simulink model "FSModem_FPGA"  (R2017b)
settings: Solver=FixedStepDiscrete  StartTime=0.0  StopTime=10.0  RelTol=1e-3
InitFcn:
  | theta = 0:pi/4:(2*pi)-(pi/4);
  | Fs_8 = cos(theta) +i*sin(theta);
  | sample_time = 1/1e6;
undefined symbols (not defined in the file): i
libraries: hdlsllib x2
settings Model: DataTypeOverride=Off  Creator=ppradhan  LastModifiedBy=ppradhan
settings DataIOCC: SaveOutput=off  SaveTime=off
settings OptimizationCC: BlockReduction=off  ConditionallyExecuteInputs=off  DefaultParameterBehavior=Inlined
settings DebuggingCC: AlgebraicLoopMsg=error  SingleTaskRateTransMsg=error  StrictBusMsg=ErrorOnBusTreatedAsVector
settings HardwareCC: ProdBitPerPointer=32  ProdBitPerSizeT=32  ProdBitPerPtrDiffT=32  ProdLargestAtomicFloat=None  ProdIntDivRoundTo=Undefined  ProdEndianess=Unspecified  ProdWordSize=32  ProdHWDeviceType=ASIC/FPGA->ASIC/FPGA  ProdEqTarget=off
settings CodeAppCC: StateflowObjectComments=on

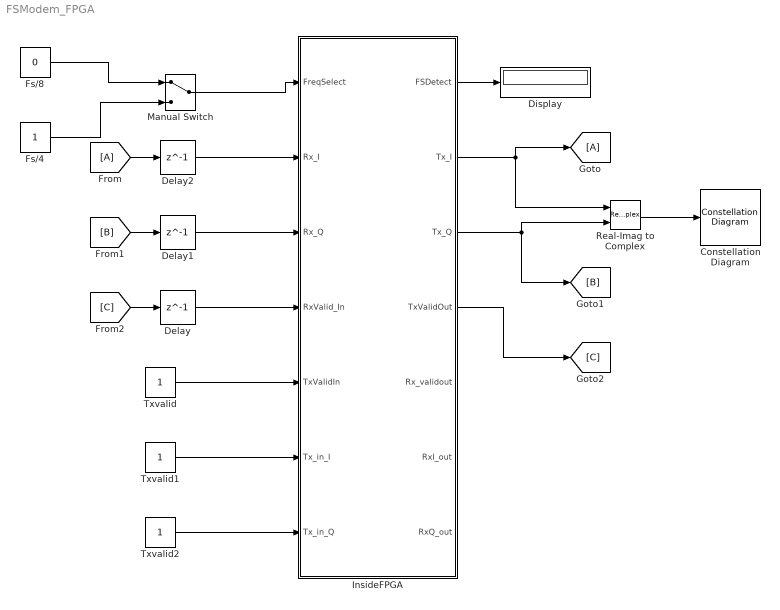
== system FSModem_FPGA ==
  Constellation Diagram : ConstellationDiagram
  Delay : Delay  DelayLength=1
  Delay1 : Delay  DelayLength=1
  Delay2 : Delay  DelayLength=1
  Display : Display
  Fs/4 : Constant  OutDataTypeStr=boolean  SampleTime=sample_time
  Fs/8 : Constant  Value=0  OutDataTypeStr=boolean  SampleTime=sample_time
  InsideFPGA : Subsystem  TreatAsAtomicUnit=on
  Manual Switch : ManualSwitch
  Real-Imag to Complex : RealImagToComplex
  Txvalid : Constant  OutDataTypeStr=boolean  SampleTime=sample_time
  Txvalid1 : Constant  OutDataTypeStr=int16  SampleTime=sample_time
  Txvalid2 : Constant  OutDataTypeStr=int16  SampleTime=sample_time
  wires:
  InsideFPGA/1(FSDetect) -> Display/1
  InsideFPGA/2(Tx_I) -> Real-Imag to Complex/1, [A]
  [A] -> Delay2/1
  InsideFPGA/3(Tx_Q) -> [B], Real-Imag to Complex/2
  [B] -> Delay1/1
  InsideFPGA/4(TxValidOut) -> [C]
  [C] -> Delay/1
  Delay/1 -> InsideFPGA/4(RxValid_In)
  Delay1/1 -> InsideFPGA/3(Rx_Q)
  Delay2/1 -> InsideFPGA/2(Rx_I)
  Real-Imag to Complex/1 -> Constellation Diagram/1
  Fs/8/1 -> Manual Switch/1
  Fs/4/1 -> Manual Switch/2
  Manual Switch/1 -> InsideFPGA/1(FreqSelect)
  Txvalid/1 -> InsideFPGA/5(TxValidIn)
  Txvalid1/1 -> InsideFPGA/6(Tx_in_I)
  Txvalid2/1 -> InsideFPGA/7(Tx_in_Q)

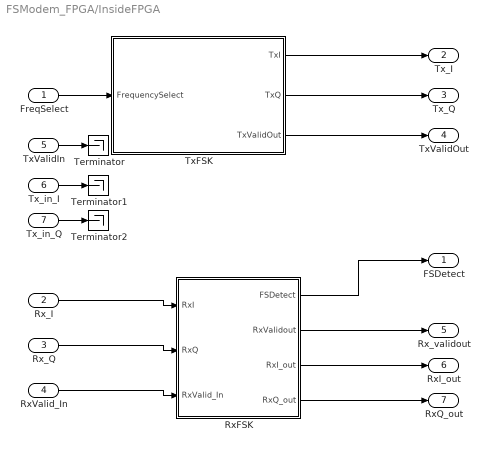
== system FSModem_FPGA/InsideFPGA ==
  FreqSelect : Inport
  Rx_I : Inport  Port=2
  Rx_Q : Inport  Port=3
  RxValid_In : Inport  Port=4
  TxValidIn : Inport  Port=5
  Tx_in_I : Inport  Port=6
  Tx_in_Q : Inport  Port=7
  RxFSK : Subsystem
  Terminator : Terminator
  Terminator1 : Terminator
  Terminator2 : Terminator
  TxFSK : Subsystem
  FSDetect : Outport
  Tx_I : Outport  Port=2
  Tx_Q : Outport  Port=3
  TxValidOut : Outport  Port=4
  Rx_validout : Outport  Port=5
  RxI_out : Outport  Port=6
  RxQ_out : Outport  Port=7
  wires:
  FreqSelect/1 -> TxFSK/1(FrequencySelect)
  RxFSK/1(FSDetect) -> FSDetect/1
  Rx_I/1 -> RxFSK/1(RxI)
  Rx_Q/1 -> RxFSK/2(RxQ)
  RxValid_In/1 -> RxFSK/3(RxValid_In)
  TxFSK/3(TxValidOut) -> TxValidOut/1
  TxFSK/1(TxI) -> Tx_I/1
  TxFSK/2(TxQ) -> Tx_Q/1
  RxFSK/2(RxValidout) -> Rx_validout/1
  TxValidIn/1 -> Terminator/1
  Tx_in_I/1 -> Terminator1/1
  Tx_in_Q/1 -> Terminator2/1
  RxFSK/3(RxI_out) -> RxI_out/1
  RxFSK/4(RxQ_out) -> RxQ_out/1

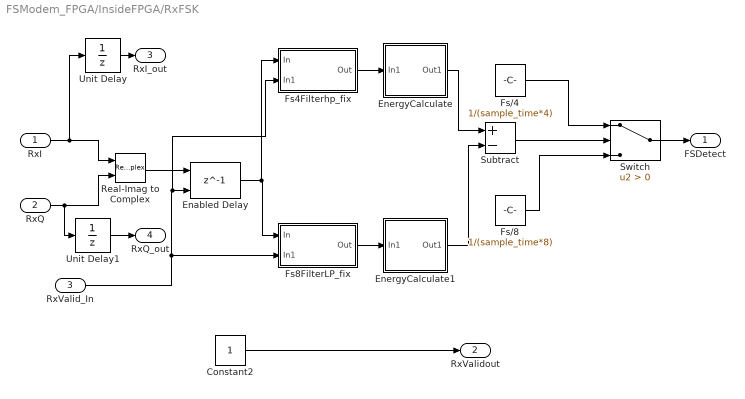
== system FSModem_FPGA/InsideFPGA/RxFSK ==
  RxI : Inport
  RxQ : Inport  Port=2
  RxValid_In : Inport  Port=3
  Constant2 : Constant  OutDataTypeStr=boolean  SampleTime=sample_time
  Enabled Delay : Delay  DelayLength=1  ShowEnablePort=on
      settings: InputPortMap=u0,e6
  EnergyCalculate : Subsystem
  EnergyCalculate1 : Subsystem
  Fs/4 : Constant  Value=1/(sample_time*4)  OutDataTypeStr=fixdt(1,16)  SampleTime=sample_time
  Fs/8 : Constant  Value=1/(sample_time*8)  OutDataTypeStr=fixdt(1,16)  SampleTime=sample_time
  Fs4Filterhp_fix : Subsystem  Tag=BlockMethodSubSystem
  Fs8FilterLP_fix : Subsystem  Tag=BlockMethodSubSystem
  Real-Imag to Complex : RealImagToComplex
  Subtract : Sum  Inputs=+-
  Switch : Switch  Criteria=u2 > Threshold
  Unit Delay : UnitDelay  SampleTime=-1
  Unit Delay1 : UnitDelay  SampleTime=-1
  FSDetect : Outport
  RxValidout : Outport  Port=2
  RxI_out : Outport  Port=3
  RxQ_out : Outport  Port=4
  wires:
  EnergyCalculate/1(Out1) -> Subtract/1
  Subtract/1 -> Switch/2
  Fs/4/1 -> Switch/1
  Fs/8/1 -> Switch/3
  Switch/1 -> FSDetect/1
  EnergyCalculate1/1(Out1) -> Subtract/2
  Fs8FilterLP_fix/1(Out) -> EnergyCalculate1/1(In1)
  Fs4Filterhp_fix/1(Out) -> EnergyCalculate/1(In1)
  RxI/1 -> Unit Delay/1, Real-Imag to Complex/1
  RxQ/1 -> Unit Delay1/1, Real-Imag to Complex/2
  Real-Imag to Complex/1 -> Enabled Delay/1
  Enabled Delay/1 -> Fs4Filterhp_fix/1(In), Fs8FilterLP_fix/1(In)
  Constant2/1 -> RxValidout/1
  RxValid_In/1 -> Fs8FilterLP_fix/2(In1), Fs4Filterhp_fix/2(In1), Enabled Delay/2
  Unit Delay/1 -> RxI_out/1
  Unit Delay1/1 -> RxQ_out/1

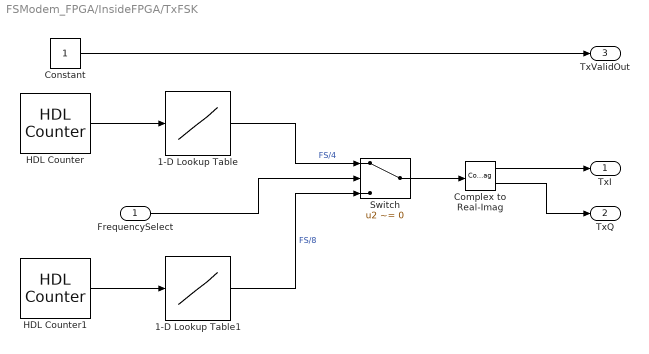
== system FSModem_FPGA/InsideFPGA/TxFSK ==
  FrequencySelect : Inport
  1-D Lookup Table : Lookup_n-D  NumberOfTableDimensions=1  BreakpointsForDimension1=[0:3]  BreakpointsForDimension1FirstPoint=10  BreakpointsForDimension2FirstPoint=10  BreakpointsForDimension1Spacing=12  BreakpointsForDimension2Spacing=12  IndexSearchMethod=Evenly spaced points  Table=[1+0*i, 0+i,-1+0*i, 0-i]  TableDataTypeStr=fixdt(1,16,14)  InterpMethod=Flat  DiagnosticForOutOfRangeInput=Error  InternalRulePriority=Speed  OutDataTypeStr=fixdt(1,16,14)  RndMeth=Simplest  InputSameDT=on
  1-D Lookup Table1 : Lookup_n-D  NumberOfTableDimensions=1  BreakpointsForDimension1=[0:7]  BreakpointsForDimension1FirstPoint=10  BreakpointsForDimension2FirstPoint=10  BreakpointsForDimension1Spacing=12  BreakpointsForDimension2Spacing=12  IndexSearchMethod=Evenly spaced points  Table=Fs_8  TableDataTypeStr=fixdt(1,16,14)  InterpMethod=Flat  DiagnosticForOutOfRangeInput=Error  InternalRulePriority=Speed  OutDataTypeStr=fixdt(1,16,14)  RndMeth=Simplest  InputSameDT=on
  Complex to Real-Imag : ComplexToRealImag
  Constant : Constant  OutDataTypeStr=boolean  SampleTime=sample_time
  HDL Counter : hdlsllib/HDL Operations/HDL Counter  CountType=Free running  CountInit=0  CountStep=1  CountMax=25  CountFromType=Initial value  CountFrom=0  CountResetPort=off  CountLoadPort=off  CountEnbPort=off  CountDirPort=off  CountDataType=Unsigned  CountWordLen=2  CountFracLen=0  CountSampTime=sample_time
      settings: SourceProductName=HDL Coder  SourceProductBaseCode=HD
  HDL Counter1 : hdlsllib/HDL Operations/HDL Counter  CountType=Free running  CountInit=0  CountStep=1  CountMax=25  CountFromType=Initial value  CountFrom=0  CountResetPort=off  CountLoadPort=off  CountEnbPort=off  CountDirPort=off  CountDataType=Unsigned  CountWordLen=3  CountFracLen=0  CountSampTime=sample_time
      settings: SourceProductName=HDL Coder  SourceProductBaseCode=HD
  Switch : Switch  Criteria=u2 ~= 0
  TxI : Outport
  TxQ : Outport  Port=2
  TxValidOut : Outport  Port=3
  wires:
  1-D Lookup Table/1 -> Switch/1  "FS/4"
  HDL Counter1/1 -> 1-D Lookup Table1/1
  FrequencySelect/1 -> Switch/2
  1-D Lookup Table1/1 -> Switch/3  "FS/8"
  HDL Counter/1 -> 1-D Lookup Table/1
  Switch/1 -> Complex to Real-Imag/1
  Complex to Real-Imag/1 -> TxI/1
  Complex to Real-Imag/2 -> TxQ/1
  Constant/1 -> TxValidOut/1

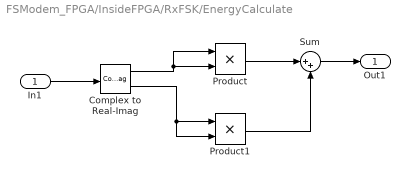
== system FSModem_FPGA/InsideFPGA/RxFSK/EnergyCalculate ==
  In1 : Inport
  Complex to Real-Imag : ComplexToRealImag
  Product : Product
  Product1 : Product
  Sum : Sum  Inputs=|++
  Out1 : Outport
  wires:
  In1/1 -> Complex to Real-Imag/1
  Complex to Real-Imag/1 -> Product/2, Product/1
  Product/1 -> Sum/1
  Complex to Real-Imag/2 -> Product1/2, Product1/1
  Product1/1 -> Sum/2
  Sum/1 -> Out1/1

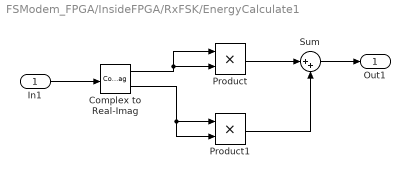
== system FSModem_FPGA/InsideFPGA/RxFSK/EnergyCalculate1 ==
  In1 : Inport
  Complex to Real-Imag : ComplexToRealImag
  Product : Product
  Product1 : Product
  Sum : Sum  Inputs=|++
  Out1 : Outport
  wires:
  Sum/1 -> Out1/1
  Product1/1 -> Sum/2
  Complex to Real-Imag/2 -> Product1/1, Product1/2
  Product/1 -> Sum/1
  Complex to Real-Imag/1 -> Product/1, Product/2
  In1/1 -> Complex to Real-Imag/1

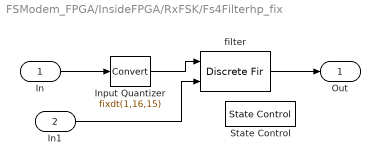
== system FSModem_FPGA/InsideFPGA/RxFSK/Fs4Filterhp_fix ==
  In : Inport
  In1 : Inport  Port=2
  Input Quantizer : DataTypeConversion  OutDataTypeStr=fixdt(1,16,15)  RndMeth=Round  SaturateOnIntegerOverflow=on
  State Control : StateControl  StateControl=Synchronous
  filter : DiscreteFir  Coefficients=[0.0013343852178826865 -0.037208942498876921 0.0096591102849806244 0.060294949982258796 0.044994895945192195 -0.096576041962710787 -0.2938256195866174 0.61241243421292701 -0.2938256195866174 -0.096576041962710787 0.044994895945192195 0.060294949982258796 0.0096591102849806244 -0.037208942498876921 0.0013343852178826865]  ShowEnablePort=on  CoefDataTypeStr=fixdt(true,16,15)  ProductDataTypeStr=fixdt(true,31,30)  AccumDataTypeStr=fixdt(true,32,30)  OutDataTypeStr=fixdt(true,16,15)  RndMeth=Convergent
      settings: InputPortMap=u0,e7
  Out : Outport
  wires:
  In/1 -> Input Quantizer/1
  Input Quantizer/1 -> filter/1
  filter/1 -> Out/1
  In1/1 -> filter/2

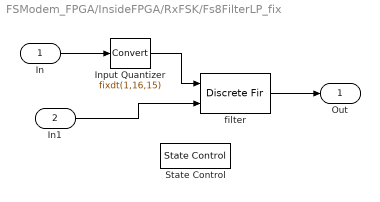
== system FSModem_FPGA/InsideFPGA/RxFSK/Fs8FilterLP_fix ==
  In : Inport
  In1 : Inport  Port=2
  Input Quantizer : DataTypeConversion  OutDataTypeStr=fixdt(1,16,15)  RndMeth=Round  SaturateOnIntegerOverflow=on
  State Control : StateControl  StateControl=Synchronous
  filter : DiscreteFir  Coefficients=[-0.0036634264370219907 -0.041218015500331405 -0.060716264187842602 -0.014844055350270549 0.12014351880942774 0.27886982134886168 0.35020150103238695 0.27886982134886168 0.12014351880942774 -0.014844055350270549 -0.060716264187842602 -0.041218015500331405 -0.0036634264370219907]  ShowEnablePort=on  CoefDataTypeStr=fixdt(true,16,16)  ProductDataTypeStr=fixdt(true,31,31)  AccumDataTypeStr=fixdt(true,33,31)  OutDataTypeStr=fixdt(true,16,15)  RndMeth=Convergent
      settings: InputPortMap=u0,e7
  Out : Outport
  wires:
  In/1 -> Input Quantizer/1
  Input Quantizer/1 -> filter/1
  filter/1 -> Out/1
  In1/1 -> filter/2
